simulink model "cable"  (R2019b)
settings: Solver=ode4  StartTime=0.0  StopTime=1  FixedStep=0.01  RelTol=1e-3
settings Model: Creator=q5461  LastModifiedBy=q5461

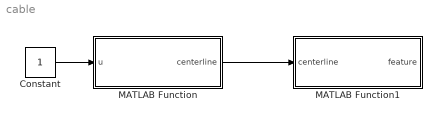
== system cable ==
  Constant : Constant
  MATLAB Function : MATLAB Function  TreatAsAtomicUnit=on
  MATLAB Function1 : MATLAB Function  TreatAsAtomicUnit=on
  wires:
  Constant/1 -> MATLAB Function/1(u)
  MATLAB Function/1(centerline) -> MATLAB Function1/1(centerline)

== matlab function cable/MATLAB Function1 ==
  data: centerline input; feature output
function feature  = fcn(centerline)
feature = zeros(14,1);
% x = zeros(50,1);
% y = zeros(50,1);
% state0 = [0.1 0 deg2rad(45)];
% state1 = [0.5 0 deg2rad(-45)];
% coder.extrinsic('dlodynamics_2D')
% [centerline,~,~] = dlodynamics_2D(state0,state1,1,[],2);
% x = 1;
% y = 1;
% x = centerline(:,1)';
% y = centerline(:,2)';
% plot(centerline(:,1),centerline(:,2))

[feature,~,~] = LSM_analytical_centerline(centerline,6,1);
end

== matlab function cable/MATLAB Function ==
  data: u input; centerline output
function centerline  = fcn(u)

centerline = zeros(50,2);
% x = zeros(50,1);
% y = zeros(50,1);
state0 = [0.1 0 deg2rad(45)];
state1 = [0.5 0 deg2rad(-45)];
coder.extrinsic('dlodynamics_2D')
[centerline,~,~] = dlodynamics_2D(state0,state1,1,[],2);
% x = 1;
% y = 1;
% x = centerline(:,1)';
% y = centerline(:,2)';
end
